simulink model "Satellite_Dynamics_V2"  (R2025b)
settings: Solver=VariableStepAuto  StartTime=0.0  StopTime=90  RelTol=1e-3
values from neighbouring files (symbols this model uses):
  initial_hw = J*Wi    [AULEsapce.m]    (also in Satellite.m)
  J = [1.10 0.05 0.00 ... (first row only)    [AULEsapce.m]    (also in Satellite.m)
  K = -lqr(A,B,Q,R)    [AULEsapce.m]    (also in Satellite.m)
  q_desired = [-0.06680 0.0481 -0.7296 -0.1385].'    [AULEsapce.m]    (also in Satellite.m)
  Qd = [-0.4078 -0.2926 -0.1687 ... (first row only)    [AULEsapce.m]    (also in Satellite.m)
  qn = sqrt(1-quaternion(1)^2-quaternion(2)^2-quaternion(3)^2)    [AULEsapce.m]    (also in Satellite.m)
  S = [0 0.2094 0.3491 ... (first row only)    [AULEsapce.m]    (also in Satellite.m)
  td = [1 0 0].'    [AULEsapce.m]    (also in Satellite.m)
  Wi = [0.1745 -0.3491 0.2094].'    [AULEsapce.m]    (also in Satellite.m)
libraries: aerolibutil x1
settings Model: Creator=mehta

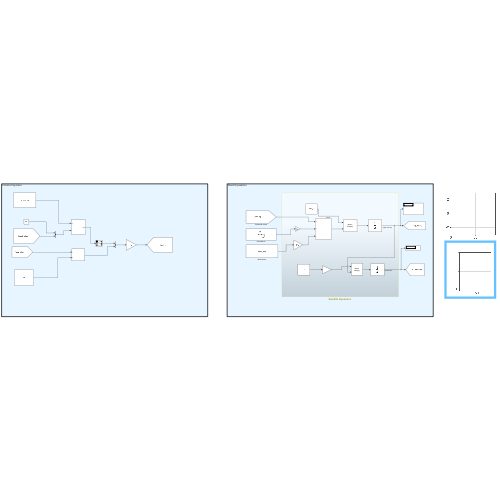
[thumbnail: Simulink's stored preview of the top-level diagram]
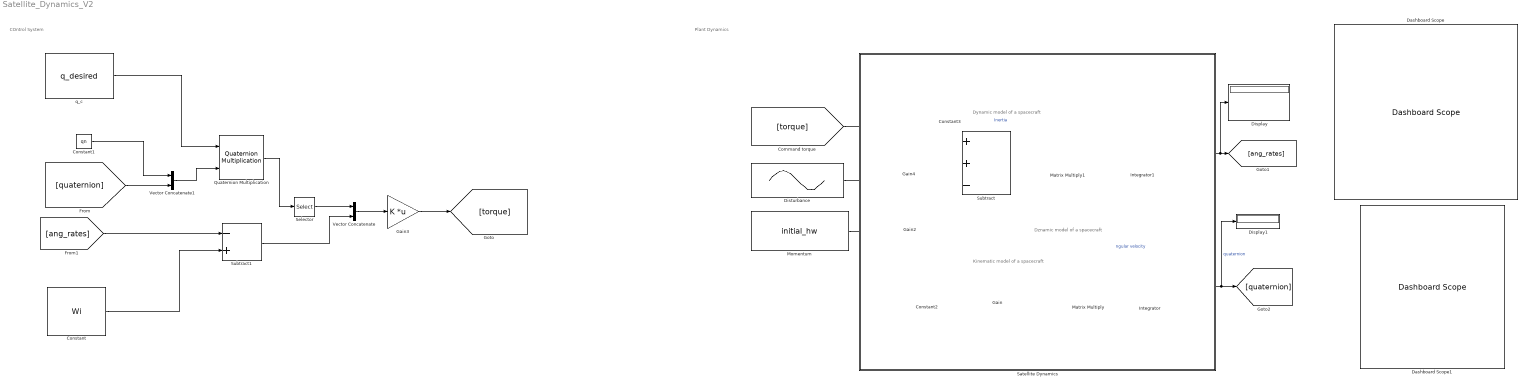
== system Satellite_Dynamics_V2 ==
  note: Dynamic model of a spacecraft
  note: Plant Dynamics
  note: Dznamic model of a spacecraft
  note: Kinematic model of a spacecraft
  note: COntrol System
  Constant : Constant  Value=Wi
  Constant1 : Constant  Value=qn
  Constant2 : Constant  Value=1/2
  Constant3 : Constant  Value=inv(J)
  Dashboard Scope : DashboardScope  FontColor=[0.0, 0.0, 0.0]
  Dashboard Scope1 : DashboardScope  FontColor=[0.0, 0.0, 0.0]
  Display : Display
  Display1 : Display
  Disturbance : Sin  Amplitude=10^(-6)  Frequency=0.1  SampleTime=0.1  VectorParams1D=off
  Gain : Gain  Gain=Qd
  Gain2 : Gain  Gain=S  Multiplication=Matrix(K*u)
  Gain3 : Gain  Gain=K  Multiplication=Matrix(K*u)
  Gain4 : Gain  Gain=td  Multiplication=Matrix(K*u)
  Integrator : Integrator
  Integrator1 : Integrator
  Matrix Multiply : Product  Multiplication=Matrix(*)
  Matrix Multiply1 : Product  Multiplication=Matrix(*)
  Momentum : Constant  Value=initial_hw
  Quaternion Multiplication : aerolibutil/Quaternion Multiplication
  "Satellite Dynamics " : Subsystem
  Selector : Selector  InputPortWidth=4  IndexOptions=Index vector (dialog)  Indices=[2 3 4]  OutputSizes=1
  Subtract : Sum  Inputs=++-
  Subtract1 : Sum  Inputs=-+
  Vector Concatenate : Concatenate
  Vector Concatenate1 : Concatenate
  q_c : Constant  Value=q_desired
  wires:
  Disturbance/1 -> Gain4/1
  Momentum/1 -> Gain2/1
  [torque] -> Subtract/1
  q_c/1 -> Quaternion Multiplication/1
  Constant2/1 -> Gain/1
  Integrator1/1 -> Matrix Multiply/2, Display/1, [ang_rates]  "ngular velocity"
  Integrator/1 -> Display1/1, [quaternion]  "quaternion"
  Matrix Multiply/1 -> Integrator/1
  Gain3/1 -> [torque]
  Quaternion Multiplication/1 -> Selector/1
  Vector Concatenate/1 -> Gain3/1
  Gain2/1 -> Subtract/3
  Gain4/1 -> Subtract/2
  Constant1/1 -> Vector Concatenate1/1
  [quaternion] -> Vector Concatenate1/2
  Selector/1 -> Vector Concatenate/1
  Matrix Multiply1/1 -> Integrator1/1
  Subtract/1 -> Matrix Multiply1/2
  Constant3/1 -> Matrix Multiply1/1  "Inertia"
  Subtract1/1 -> Vector Concatenate/2
  [ang_rates] -> Subtract1/1
  Constant/1 -> Subtract1/2
  Gain/1 -> Matrix Multiply/1
  Vector Concatenate1/1 -> Quaternion Multiplication/2

== system Satellite_Dynamics_V2/Satellite Dynamics  ==
  note: Satellite Dynamics Block:
